simulink model "PTOSwt_VD"  (R2016b)
settings: configuration reference "CodeGenConfigSet" (kept outside this file)
values from neighbouring files (symbols this model uses):
  MoFPTO_uThresCalMsgA_CA = Calibration.Parameter    [init_PTOSwt_VD.m]    (also in init_PTOSwt_VD_SIL.m = Simulink.Parameter)
  PTOSwt_bDfl_C = Calibration.Parameter    [init_PTOSwt_VD.m]    (also in init_PTOSwt_VD_SIL.m = Simulink.Parameter)
  PTOSwt_bEnblSwt_C = Calibration.Parameter    [init_PTOSwt_VD.m]    (also in init_PTOSwt_VD_SIL.m = Simulink.Parameter)
  PTOSwt_stDfl_C = Calibration.Parameter    [init_PTOSwt_VD.m]    (also in init_PTOSwt_VD_SIL.m = Simulink.Parameter)
  SigTst_stPTOSwt = Calibration.Parameter    [init_PTOSwt_VD.m]    (also in init_PTOSwt_VD_SIL.m = Simulink.Parameter)
  SigTst_swtPTOSwt = Calibration.Parameter    [init_PTOSwt_VD.m]    (also in init_PTOSwt_VD_SIL.m = Simulink.Parameter)
undefined symbols (not defined in the file or in its folder): Switch_conv
settings Model: Creator=lenovo  LastModifiedBy=bianxuyin
settings ConfigSetRef: SourceLocation=Base Workspace

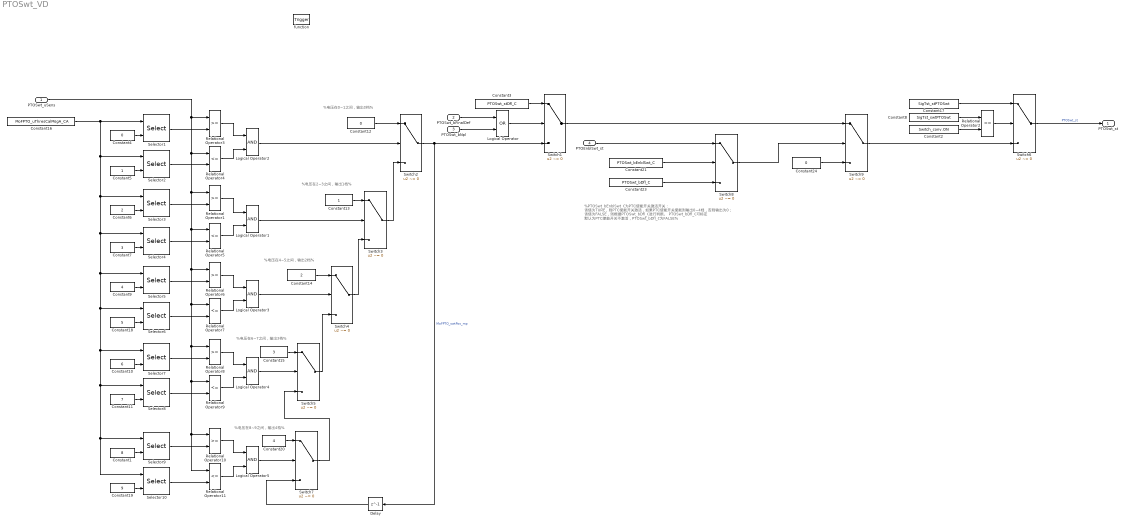
== system PTOSwt_VD ==
  note: %电压在6~7之间，输出3档%
  note: %电压在4~5之间，输出2档%
  note: %电压在2~3之间，输出1档%
  note: %电压在0~1之间，输出0档%
  note: %电压在8~9之间，输出4档%
  note: %PTOSwt_bEnblSwt_C为PTO使能开关激活开关：
      | 该值为TURE，则PTO使能开关激活，如果PTO使能开关使能则输出0~4档，否则输出为0；
      | 该值为FALSE，则根据PTOSwt_bDfl_C进行判断。
      |
      |  PTOSwt_bDfl_C可标定
      |
      | 默认为PTO使能开关不激活，PTOSwt_bDfl_C为FALSE%
  PTOSwt_uSens : Inport  Tag=mv  Description=Sensed value of multiple state switch  OutMin=0  OutMax=5000  OutDataTypeStr=Ad_mv
  PTOSwt_bFinalDef : Inport  Description=PTO switch sensor SRC finally defect flag  Port=2  OutMin=0  OutMax=1  OutDataTypeStr=boolean
  PTOSwt_bNpl : Inport  Description=PTO switch sensor non plausible flag  Port=3  OutMin=0  OutMax=1  OutDataTypeStr=boolean
  PTOEnblSwt_st : Inport  Description=PTO enable switch status  Port=4  OutMin=0  OutMax=1  OutDataTypeStr=boolean
  function : TriggerPort  TriggerType=function-call  VariantControl=Variant
  Constant1 : Constant  Value=8  OutDataTypeStr=uint8
  Constant10 : Constant  Value=6  OutDataTypeStr=uint8
  Constant11 : Constant  Value=7  OutDataTypeStr=uint8
  Constant12 : Constant  RequirementInfo={'other' 'APP_requirements.doc' '@Simulink_requirement_item_28' 'true' '油门保护模式' '' } %GIDa_893ab110_c936_4738_8d67_daf0700ea0a1  Value=0  OutDataTypeStr=uint8
  Constant13 : Constant  RequirementInfo={'other' 'APP_requirements.doc' '@Simulink_requirement_item_28' 'true' '油门保护模式' '' } %GIDa_34e7425b_5d79_47ff_95cb_d0785d1d5830  OutDataTypeStr=uint8
  Constant14 : Constant  RequirementInfo={'other' 'APP_requirements.doc' '@Simulink_requirement_item_28' 'true' '油门保护模式' '' } %GIDa_0e89e2df_c72a_43aa_8d39_5567396a794a  Value=2  OutDataTypeStr=uint8
  Constant15 : Constant  RequirementInfo={'other' 'APP_requirements.doc' '@Simulink_requirement_item_28' 'true' '油门保护模式' '' } %GIDa_b791964d_f37f_4375_8388_08e5f9a2d0d9  Value=3  OutDataTypeStr=uint8
  Constant16 : Constant  Value=MoFPTO_uThresCalMsgA_CA
  Constant17 : Constant  RequirementInfo={'other' 'APP_requirements.doc' '@Simulink_requirement_item_28' 'true' '油门保护模式' '' } %GIDa_f46c813f_52d1_47bb_ad84_937ab842d653  Value=SigTst_stPTOSwt
  Constant18 : Constant  Value=5  OutDataTypeStr=uint8
  Constant19 : Constant  Value=9  OutDataTypeStr=uint8
  Constant2 : Constant  RequirementInfo={'other' 'APP_requirements.doc' '@Simulink_requirement_item_28' 'true' '油门保护模式' '' } %GIDa_7f837fd2_cd73_481f_8248_f37f4a512480  Value=Switch_conv.ON  OutDataTypeStr=Inherit: Inherit via back propagation
  Constant20 : Constant  RequirementInfo={'other' 'APP_requirements.doc' '@Simulink_requirement_item_28' 'true' '油门保护模式' '' } %GIDa_b8983774_e14e_43aa_88c7_9cd603d5a9bf  Value=4  OutDataTypeStr=uint8
  Constant21 : Constant  RequirementInfo={'other' 'APP_requirements.doc' '@Simulink_requirement_item_28' 'true' '油门保护模式' '' } %GIDa_b7df32f1_d4c8_46b7_ada2_c816cbfb88f6  Value=PTOSwt_bEnblSwt_C
  Constant23 : Constant  RequirementInfo={'other' 'APP_requirements.doc' '@Simulink_requirement_item_28' 'true' '油门保护模式' '' } %GIDa_bb2ef586_8640_4f44_86e4_1d375fd16b21  Value=PTOSwt_bDfl_C
  Constant24 : Constant  RequirementInfo={'other' 'APP_requirements.doc' '@Simulink_requirement_item_28' 'true' '油门保护模式' '' } %GIDa_8c7169e7_3fbb_49b8_b096_0ef4024ff1e6  Value=0  OutDataTypeStr=uint8
  Constant3 : Constant  RequirementInfo={'other' 'APP_requirements.doc' '@Simulink_requirement_item_28' 'true' '油门保护模式' '' } %GIDa_15aa0d73_13cc_40ab_85e1_637fb13eb815  Value=PTOSwt_stDfl_C
  Constant4 : Constant  Value=0  OutDataTypeStr=uint8
  Constant5 : Constant  OutDataTypeStr=uint8
  Constant6 : Constant  Value=2  OutDataTypeStr=uint8
  Constant7 : Constant  Value=3  OutDataTypeStr=uint8
  Constant8 : Constant  RequirementInfo={'other' 'APP_requirements.doc' '@Simulink_requirement_item_28' 'true' '油门保护模式' '' } %GIDa_593ef5a6_e70c_4188_9cb4_3964b3e2d54b  Value=SigTst_swtPTOSwt
  Constant9 : Constant  Value=4  OutDataTypeStr=uint8
  Delay : Delay  DelayLength=1  InitialCondition=0
  Logical Operator : Logic  Operator=OR  AllPortsSameDT=off  OutDataTypeStr=boolean
  Logical Operator{1..5} (5 alike) : Logic  AllPortsSameDT=off  OutDataTypeStr=boolean
  Relational Operator{1,3,6,8,10} (5 alike) : RelationalOperator  OutDataTypeStr=boolean  RndMeth=Nearest  InputSameDT=on
  Relational Operator{4..5,7,9,11} (5 alike) : RelationalOperator  Operator=<=  OutDataTypeStr=boolean  RndMeth=Nearest  InputSameDT=on
  Relational Operator2 : RelationalOperator  RequirementInfo={'other' 'APP_requirements.doc' '@Simulink_requirement_item_28' 'true' '油门保护模式' '' } %GIDa_143eae70_627f_4269_b7f9_9d7e45b9ec8b  Operator===  OutDataTypeStr=boolean  RndMeth=Nearest  InputSameDT=on
  Selector{1..10} (10 alike) : Selector  IndexMode=Zero-based  InputPortWidth=10  IndexOptions=Index vector (port)  Indices=[1 3]  OutputSizes=1
  Switch{1..9} (9 alike) : Switch  Criteria=u2 ~= 0  InputSameDT=on
  PTOSwt_st : Outport  Description=Power Take-off switch current state for a specific input voltage  OutMin=0  OutMax=255  OutDataTypeStr=State_uint8
  wires:
  Switch2/1 -> Delay/1, Switch1/3  "MoFPTO_swtPos_mp"
  Switch3/1 -> Switch2/3
  Switch5/1 -> Switch4/3
  Switch4/1 -> Switch3/3
  Logical Operator4/1 -> Switch5/2
  Constant14/1 -> Switch4/1
  Logical Operator3/1 -> Switch4/2
  Constant13/1 -> Switch3/1
  Logical Operator1/1 -> Switch3/2
  Constant12/1 -> Switch2/1
  Constant15/1 -> Switch5/1
  Logical Operator2/1 -> Switch2/2
  Switch6/1 -> PTOSwt_st/1  "PTOSwt_st"
  Constant7/1 -> Selector4/2
  Relational Operator7/1 -> Logical Operator3/2
  PTOSwt_bNpl/1 -> Logical Operator/2
  Selector8/1 -> Relational Operator9/2
  Relational Operator6/1 -> Logical Operator3/1
  Constant6/1 -> Selector3/2
  Relational Operator8/1 -> Logical Operator4/1
  Selector7/1 -> Relational Operator8/2
  Logical Operator/1 -> Switch1/2
  Relational Operator9/1 -> Logical Operator4/2
  Constant9/1 -> Selector5/2
  Constant10/1 -> Selector7/2
  Constant11/1 -> Selector8/2
  Selector4/1 -> Relational Operator5/2
  Relational Operator5/1 -> Logical Operator1/2
  Relational Operator1/1 -> Logical Operator1/1
  Selector5/1 -> Relational Operator6/2
  Selector3/1 -> Relational Operator1/2
  Constant8/1 -> Relational Operator2/1
  Constant17/1 -> Switch6/1
  Constant2/1 -> Relational Operator2/2
  Relational Operator2/1 -> Switch6/2
  Relational Operator4/1 -> Logical Operator2/2
  Relational Operator3/1 -> Logical Operator2/1
  Constant5/1 -> Selector2/2
  PTOSwt_bFinalDef/1 -> Logical Operator/1
  Constant3/1 -> Switch1/1
  Constant4/1 -> Selector1/2
  Selector1/1 -> Relational Operator3/2
  Constant18/1 -> Selector6/2
  Selector2/1 -> Relational Operator4/2
  Selector6/1 -> Relational Operator7/2
  Constant16/1 -> Selector1/1, Selector2/1, Selector3/1, Selector4/1, Selector5/1, Selector6/1, Selector10/1, Selector9/1, Selector8/1, Selector7/1
  Selector10/1 -> Relational Operator11/2
  PTOSwt_uSens/1 -> Relational Operator3/1, Relational Operator4/1, Relational Operator1/1, Relational Operator5/1, Relational Operator6/1, Relational Operator7/1, Relational Operator10/1, Relational Operator11/1, Relational Operator9/1, Relational Operator8/1
  Relational Operator10/1 -> Logical Operator5/1
  Selector9/1 -> Relational Operator10/2
  Relational Operator11/1 -> Logical Operator5/2
  Constant1/1 -> Selector9/2
  Constant19/1 -> Selector10/2
  Constant20/1 -> Switch7/1
  Switch7/1 -> Switch5/3
  Logical Operator5/1 -> Switch7/2
  Delay/1 -> Switch7/3
  Switch8/1 -> Switch9/2
  Switch1/1 -> Switch9/1
  Constant24/1 -> Switch9/3
  Switch9/1 -> Switch6/3
  Constant23/1 -> Switch8/3
  PTOEnblSwt_st/1 -> Switch8/1
  Constant21/1 -> Switch8/2
